simulink model "task4"  (R2022b)
settings: Solver=VariableStepAuto  StartTime=0.0  StopTime=stoptime  RelTol=1e-9
values from neighbouring files (symbols this model uses):
  I = diag(I)    [task6main.m]
  I_inv = pinv(I)    [task6main.m]
  Ir = 0.005    [task6main.m]
  k = [0;0;1]    [task6main.m]
  M = [0;0;0]    [task6main.m]
  Mr = 0    [task6main.m]
  w0 = cat(1,w0,wr0)    [task6main.m]
libraries: matrix_library x1
settings Model: Creator=a1pab  LastModifiedBy=a1pab

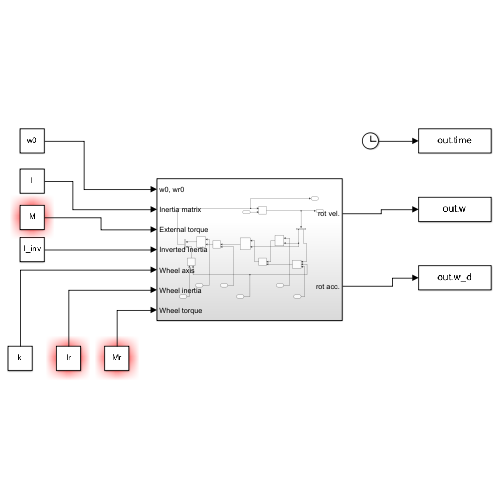
[thumbnail: Simulink's stored preview of the top-level diagram]
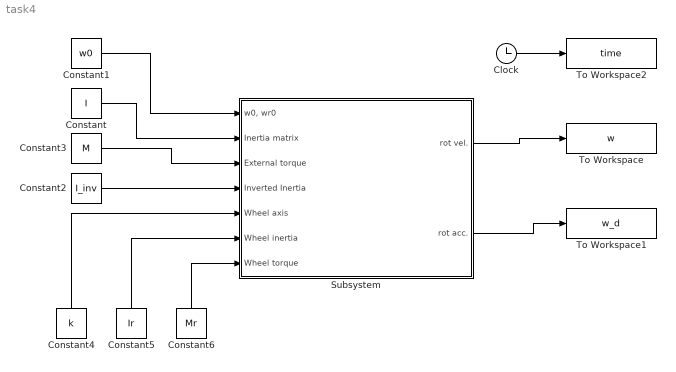
== system task4 ==
  Clock : Clock
  Constant : Constant  Value=I  VectorParams1D=off
  Constant1 : Constant  Value=w0  VectorParams1D=off
  Constant2 : Constant  Value=I_inv  VectorParams1D=off
  Constant3 : Constant  Value=M  VectorParams1D=off
  Constant4 : Constant  Value=k  VectorParams1D=off
  Constant5 : Constant  Value=Ir
  Constant6 : Constant  Value=Mr
  Subsystem : Subsystem
  To Workspace : ToWorkspace  VariableName=w  SampleTime=-1
  To Workspace1 : ToWorkspace  VariableName=w_d  SampleTime=-1
  To Workspace2 : ToWorkspace  VariableName=time  SampleTime=-1
  wires:
  Subsystem/1(rot vel.) -> To Workspace/1
  Subsystem/2(rot acc.) -> To Workspace1/1
  Constant/1 -> Subsystem/2(Inertia matrix)
  Constant1/1 -> Subsystem/1("w0, wr0")
  Clock/1 -> To Workspace2/1
  Constant2/1 -> Subsystem/4(Inverted Inertia)
  Constant3/1 -> Subsystem/3(External torque)
  Constant4/1 -> Subsystem/5(Wheel axis)
  Constant6/1 -> Subsystem/7(Wheel torque)
  Constant5/1 -> Subsystem/6(Wheel inertia)

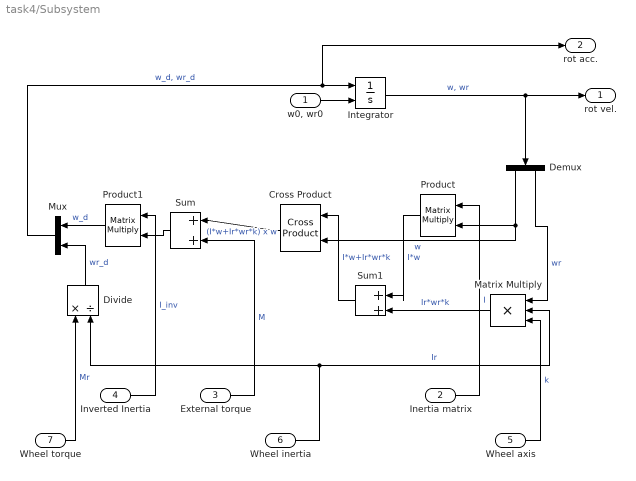
== system task4/Subsystem ==
  "w0, wr0" : Inport
  Inertia matrix : Inport  Port=2
  External torque : Inport  Port=3
  Inverted Inertia : Inport  Port=4
  Wheel axis : Inport  Port=5
  Wheel inertia : Inport  Port=6
  Wheel torque : Inport  Port=7
  Cross Product : matrix_library/Cross Product
  Demux : Demux  Outputs=2
  Divide : Product  Inputs=*/
  Integrator : Integrator  InitialConditionSource=external
  Matrix Multiply : Product  Inputs=3
  Mux : Mux  Inputs=2
  Product : Product  Multiplication=Matrix(*)
  Product1 : Product  Multiplication=Matrix(*)
  Sum : Sum  Inputs=|++
  Sum1 : Sum  Inputs=|++
  rot vel. : Outport
  rot acc. : Outport  Port=2
  wires:
  Mux/1 -> rot acc./1, Integrator/1  "w_d, wr_d"
  Integrator/1 -> Demux/1, rot vel./1  "w, wr"
  "w0, wr0"/1 -> Integrator/2
  Product/1 -> Sum1/1  "I*w"
  Cross Product/1 -> Sum/1  "(I*w+Ir*wr*k) x w"
  Inverted Inertia/1 -> Product1/1  "I_inv"
  Inertia matrix/1 -> Product/1  "I"
  Sum/1 -> Product1/2
  External torque/1 -> Sum/2  "M"
  Product1/1 -> Mux/1  "w_d"
  Wheel torque/1 -> Divide/1  "Mr"
  Wheel inertia/1 -> Matrix Multiply/2, Divide/2  "Ir"
  Divide/1 -> Mux/2  "wr_d"
  Demux/1 -> Cross Product/2, Product/2  "w"
  Sum1/1 -> Cross Product/1  "I*w+Ir*wr*k"
  Demux/2 -> Matrix Multiply/1  "wr"
  Matrix Multiply/1 -> Sum1/2  "Ir*wr*k"
  Wheel axis/1 -> Matrix Multiply/3  "k"
